simulink model "ControleNL_Degrau_2020a"  (R2020a)
settings: Solver=FixedStepAuto  StartTime=0  StopTime=10  FixedStep=1e-3  RelTol=1e-3
values from neighbouring files (symbols this model uses):
  alpha = alpha_vec(l)    [kermani_parameters.m]    (also in teste_controle_nao_linear.m = 0.1)
  Fc = Fc_vec(k)    [kermani_parameters.m]    (also in teste_controle_nao_linear.m = 0.5)
  Fs = Fs_vec(j)    [kermani_parameters.m]    (also in teste_controle_nao_linear.m = 1.5)
  Jeff = 0.5    [kermani_parameters.m]    (also in teste_controle_nao_linear.m)
  K = (90/12)*(2*pi/60)    (= 0.785398163397)    [kermani_parameters.m]    (also in teste_controle_nao_linear.m)
  Kd = (2*xi*wn*Jeff - Beff)/K    (= 17.8253536263)    [kermani_parameters.m]    (also in teste_controle_nao_linear.m = -44.5633840657)
  Kp = (wn^2*Jeff)/K    (= 143.239448783)    [kermani_parameters.m]    (also in teste_controle_nao_linear.m)
  N = 3    [kermani_parameters.m]    (also in teste_controle_nao_linear.m)
  r = 1./[231.22*4 139.138 139.138 231.22 231.22]    [kermani_parameters.m]    (also in teste_controle_nao_linear.m)
  sigma0 = sigma0_vec(m)    [kermani_parameters.m]    (also in teste_controle_nao_linear.m = 10000)
  sigma1 = sigma1_vec(n)    [kermani_parameters.m]    (also in teste_controle_nao_linear.m = 500)
  sigma2 = sigma2_vec(o)    [kermani_parameters.m]    (also in teste_controle_nao_linear.m = 50)
libraries: simulink_extras x5
(part 1 of 2)
settings Model: Creator=Karoline  LastModifiedBy=lunet
settings DataIOCC: ReturnWorkspaceOutputs=off
settings DebuggingCC: ArithmeticOperatorsInVariantConditions=warning
settings SFSimCC: SimUseLocalCustomCode=off  CustomCodeUndefinedFunction=UseInterfaceOnly
settings RTWCC: RTWUseLocalCustomCode=off
settings CodeAppCC: StateflowObjectComments=on

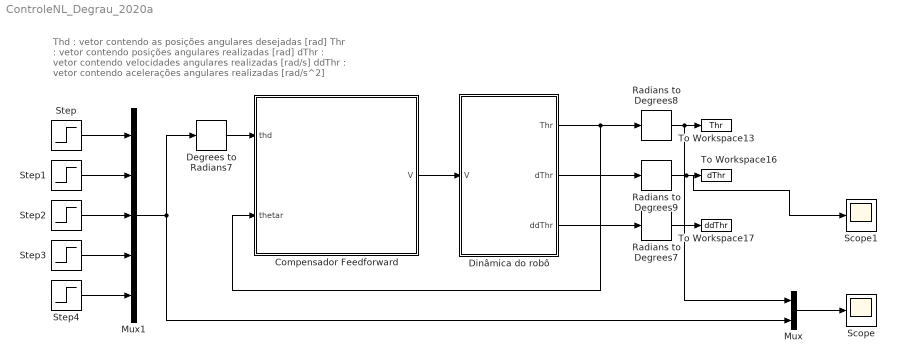
== system ControleNL_Degrau_2020a ==
  note: Thd : vetor contendo as posições angulares desejadas [rad]
      | Thr : vetor contendo posições angulares realizadas [rad]
      | dThr : vetor contendo velocidades angulares realizadas [rad/s]
      | ddThr : vetor contendo acelerações angulares realizadas [rad/s^2]
  Compensador Feedforward : Subsystem
  Degrees to Radians7 : simulink_extras/Transformations/Degrees to Radians
  Dinâmica do robô : Subsystem
  Mux : Mux  Inputs=2
  Mux1 : Mux  Inputs=5
  Radians to Degrees7 : simulink_extras/Transformations/Radians to Degrees
  Radians to Degrees8 : simulink_extras/Transformations/Radians to Degrees
  Radians to Degrees9 : simulink_extras/Transformations/Radians to Degrees
  Scope : Scope
  Scope1 : Scope
  Step : Step  After=10  SampleTime=0
  Step{1..4} (4 alike) : Step  After=0  SampleTime=0
  To Workspace13 : ToWorkspace  VariableName=Thr  SaveFormat=Structure With Time  SampleTime=-1
  To Workspace16 : ToWorkspace  VariableName=dThr  SaveFormat=Structure With Time  SampleTime=-1
  To Workspace17 : ToWorkspace  VariableName=ddThr  SaveFormat=Structure With Time  SampleTime=-1
  wires:
  Radians to Degrees9/1 -> Scope1/1, To Workspace16/1
  Radians to Degrees8/1 -> Mux/1, To Workspace13/1
  Radians to Degrees7/1 -> To Workspace17/1
  Dinâmica do robô/3(ddThr) -> Radians to Degrees7/1
  Dinâmica do robô/1(Thr) -> Compensador Feedforward/2(thetar), Radians to Degrees8/1
  Compensador Feedforward/1(V) -> Dinâmica do robô/1(V)
  Degrees to Radians7/1 -> Compensador Feedforward/1(thd)
  Dinâmica do robô/2("dThr ") -> Radians to Degrees9/1
  Mux/1 -> Scope/1
  Step/1 -> Mux1/1
  Step1/1 -> Mux1/2
  Step2/1 -> Mux1/3
  Step3/1 -> Mux1/4
  Step4/1 -> Mux1/5
  Mux1/1 -> Mux/2, Degrees to Radians7/1

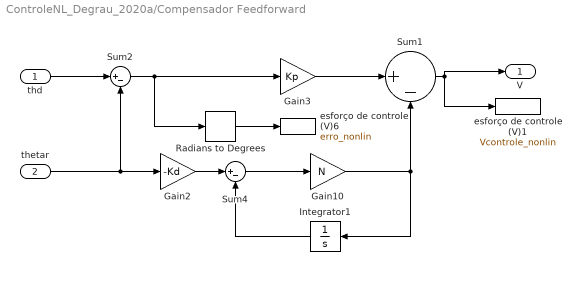
== system ControleNL_Degrau_2020a/Compensador Feedforward ==
  thd : Inport
  thetar : Inport  Port=2
  Gain10 : Gain  Gain=N
  Gain2 : Gain  Gain=-Kd
  Gain3 : Gain  Gain=Kp
  Integrator1 : Integrator
  Radians to Degrees : simulink_extras/Transformations/Radians to Degrees
  Sum1 : Sum  Inputs=|+-
  Sum2 : Sum  Inputs=|+-
  Sum4 : Sum  Inputs=|+-
  esforço de controle (V)1 : ToWorkspace  VariableName=Vcontrole_nonlin  SaveFormat=Structure With Time  SampleTime=-1
  esforço de controle (V)6 : ToWorkspace  VariableName=erro_nonlin  SaveFormat=Structure With Time  SampleTime=-1
  V : Outport  VectorParamsAs1DForOutWhenUnconnected=off
  wires:
  Gain2/1 -> Sum4/1
  thetar/1 -> Sum2/2, Gain2/1
  Sum4/1 -> Gain10/1
  Integrator1/1 -> Sum4/2
  Gain10/1 -> Sum1/2, Integrator1/1
  thd/1 -> Sum2/1
  Gain3/1 -> Sum1/1
  Sum1/1 -> V/1, esforço de controle (V)1/1
  Radians to Degrees/1 -> esforço de controle (V)6/1
  Sum2/1 -> Radians to Degrees/1, Gain3/1

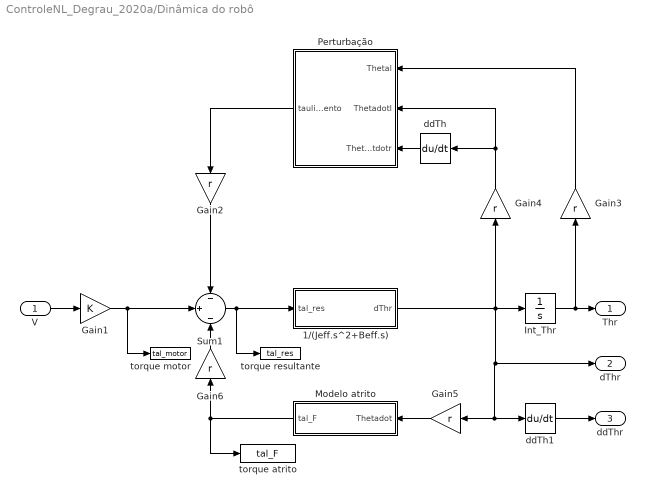
== system ControleNL_Degrau_2020a/Dinâmica do robô ==
  V : Inport
  1/(Jeff.s^2+Beff.s) : Subsystem
  Gain1 : Gain  Gain=K
  Gain{2..6} (5 alike) : Gain  Gain=r
  Int_Thr : Integrator  Tag=Int_Thr  InitialCondition=[0 0 0 0 0]
  Modelo atrito : Subsystem
  Perturbação : Subsystem
  Sum1 : Sum  Inputs=-|+|-
  ddTh : Derivative
  ddTh1 : Derivative
  torque atrito : ToWorkspace  VariableName=tal_F  SaveFormat=Structure With Time  SampleTime=-1
  torque motor : ToWorkspace  VariableName=tal_motor  SaveFormat=Structure With Time  SampleTime=-1
  torque resultante : ToWorkspace  VariableName=tal_res  SaveFormat=Structure With Time  SampleTime=-1
  Thr : Outport  VectorParamsAs1DForOutWhenUnconnected=off
  "dThr " : Outport  Port=2  VectorParamsAs1DForOutWhenUnconnected=off
  ddThr : Outport  Port=3  VectorParamsAs1DForOutWhenUnconnected=off
  wires:
  Perturbação/1(tauligamento) -> Gain2/1
  Gain1/1 -> torque motor/1, Sum1/2
  Int_Thr/1 -> Thr/1, Gain3/1
  V/1 -> Gain1/1
  Gain2/1 -> Sum1/1
  ddTh/1 -> Perturbação/3(Thetadotdotr)
  Gain3/1 -> Perturbação/1(Thetal)
  Gain4/1 -> ddTh/1, Perturbação/2(Thetadotl)
  Sum1/1 -> torque resultante/1, 1/(Jeff.s^2+Beff.s)/1(tal_res)
  ddTh1/1 -> ddThr/1
  1/(Jeff.s^2+Beff.s)/1(dThr) -> Gain5/1, ddTh1/1, "dThr "/1, Gain4/1, Int_Thr/1
  Modelo atrito/1(tal_F) -> torque atrito/1, Gain6/1
  Gain5/1 -> Modelo atrito/1(Thetadot)
  Gain6/1 -> Sum1/3

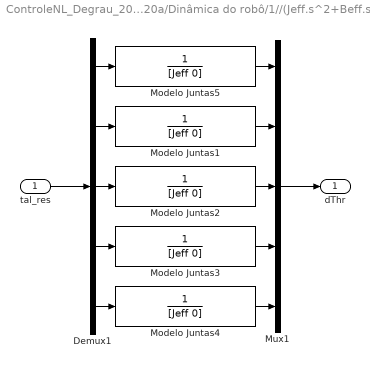
== system ControleNL_Degrau_2020a/Dinâmica do robô/1//(Jeff.s^2+Beff.s) ==
  tal_res : Inport
  Demux1 : Demux  Outputs=5
  Modelo Juntas{1..5} (5 alike) : TransferFcn  Denominator=[Jeff 0]
  Mux1 : Mux  Inputs=5
  dThr : Outport
  wires:
  Modelo Juntas5/1 -> Mux1/1
  Demux1/1 -> Modelo Juntas5/1
  Mux1/1 -> dThr/1
  tal_res/1 -> Demux1/1
  Demux1/2 -> Modelo Juntas1/1
  Modelo Juntas1/1 -> Mux1/2
  Demux1/5 -> Modelo Juntas4/1
  Demux1/4 -> Modelo Juntas3/1
  Demux1/3 -> Modelo Juntas2/1
  Modelo Juntas2/1 -> Mux1/3
  Modelo Juntas3/1 -> Mux1/4
  Modelo Juntas4/1 -> Mux1/5

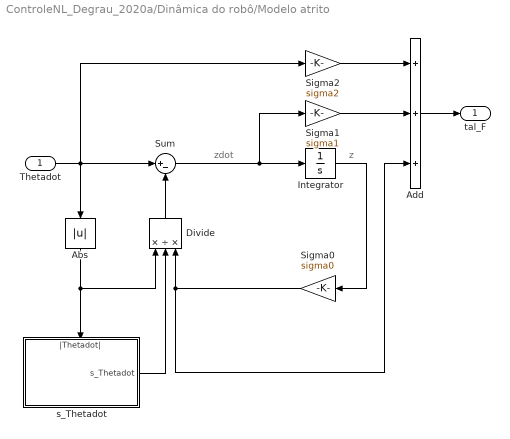
== system ControleNL_Degrau_2020a/Dinâmica do robô/Modelo atrito ==
  note: z
  note: zdot
  Thetadot : Inport
  Abs : Abs
  Add : Sum  Inputs=+++
  Divide : Product  Inputs=*/*
  Integrator : Integrator
  Sigma0 : Gain  Gain=sigma0
  Sigma1 : Gain  Gain=sigma1
  Sigma2 : Gain  Gain=sigma2
  Sum : Sum  Inputs=|+-
  s_Thetadot : Subsystem
      settings: PortSchema="{\"entries\":[{\"content\":{\"sides\":[{\"content\":{\"connectorIds\":[]},\"type\":\"ConnectorPlacement.EquallySpacedRectSide\",\"uuid\":\"4c4b190b-c928-4253-93d1-fd2ae137e0ab\"},{\"content\":{\"connectorIds\":[\"Out1\"],\"side\":\"RIGHT\"},\"type\":\"ConnectorPlacement.EquallySpacedRectSide\",\"uuid\":\"6a4109ad-b0a7-44dc-94f8-84112378c3da\"},{\"content\":{\"connectorIds\":[\"In1\"],\"side\":\"TOP\"},\"type\":\"ConnectorPlacement.EquallySpacedRectSide\",\"uuid\":\"364d9b06-17df-4fa5-ae25-87ed6816814d\"}]},\"type\":\"ConnectorPlacement.EquallySpacedConnector\",\"uuid\":\"c598e9c2-b687-45ab-b3d0-f2b281a49fb7\"}],\"packageUris\":[\"http://schema.mathworks.com/mf0/Connector/19700101\"],\"version\":\"1.0\"}"
  tal_F : Outport
  wires:
  Sigma0/1 -> Divide/3, Add/3
  Sigma1/1 -> Add/2
  Divide/1 -> Sum/2
  Abs/1 -> s_Thetadot/1(|Thetadot|), Divide/1
  s_Thetadot/1(s_Thetadot) -> Divide/2
  Sum/1 -> Sigma1/1, Integrator/1
  Thetadot/1 -> Sigma2/1, Sum/1, Abs/1
  Sigma2/1 -> Add/1
  Integrator/1 -> Sigma0/1
  Add/1 -> tal_F/1

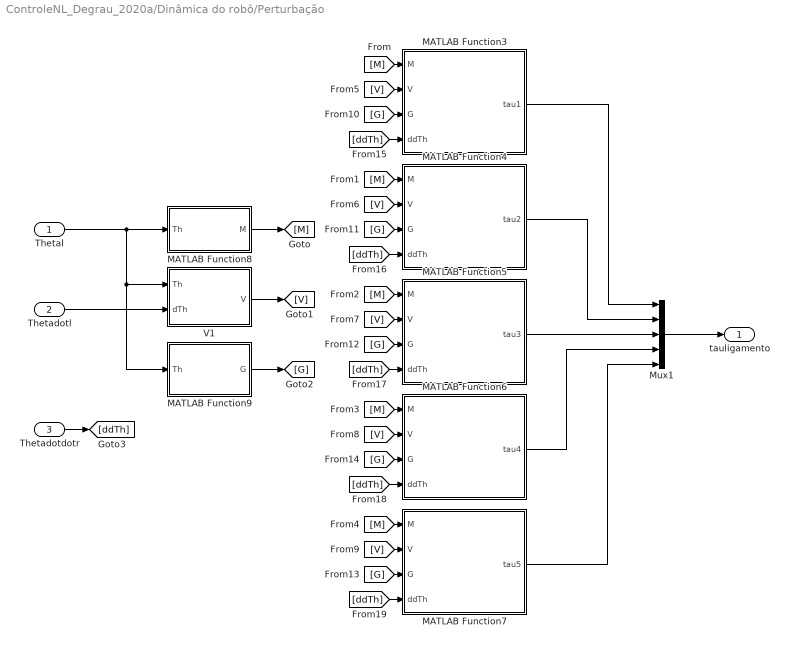
== system ControleNL_Degrau_2020a/Dinâmica do robô/Perturbação ==
  Thetal : Inport
  Thetadotl : Inport  Port=2
  Thetadotdotr : Inport  Port=3
  MATLAB Function3 : MATLAB Function  TreatAsAtomicUnit=on
  MATLAB Function4 : MATLAB Function  TreatAsAtomicUnit=on
  MATLAB Function5 : MATLAB Function  TreatAsAtomicUnit=on
  MATLAB Function6 : MATLAB Function  TreatAsAtomicUnit=on
  MATLAB Function7 : MATLAB Function  TreatAsAtomicUnit=on
  MATLAB Function8 : MATLAB Function  TreatAsAtomicUnit=on
  MATLAB Function9 : MATLAB Function  TreatAsAtomicUnit=on
  Mux1 : Mux  Inputs=5
  V1 : MATLAB Function  TreatAsAtomicUnit=on
  tauligamento : Outport  VectorParamsAs1DForOutWhenUnconnected=off
  wires:
  [G] -> MATLAB Function6/3(G)
  MATLAB Function8/1(M) -> [M]
  [M] -> MATLAB Function6/1(M)
  [M] -> MATLAB Function4/1(M)
  [M] -> MATLAB Function3/1(M)
  Thetal/1 -> MATLAB Function8/1(Th), MATLAB Function9/1(Th), V1/1(Th)
  [ddTh] -> MATLAB Function5/4(ddTh)
  [V] -> MATLAB Function3/2(V)
  [ddTh] -> MATLAB Function3/4(ddTh)
  [G] -> MATLAB Function7/3(G)
  [ddTh] -> MATLAB Function6/4(ddTh)
  [V] -> MATLAB Function6/2(V)
  Thetadotl/1 -> V1/2(dTh)
  [G] -> MATLAB Function5/3(G)
  [G] -> MATLAB Function3/3(G)
  [G] -> MATLAB Function4/3(G)
  MATLAB Function9/1(G) -> [G]
  [V] -> MATLAB Function7/2(V)
  [ddTh] -> MATLAB Function4/4(ddTh)
  [V] -> MATLAB Function5/2(V)
  [V] -> MATLAB Function4/2(V)
  V1/1(V) -> [V]
  [M] -> MATLAB Function7/1(M)
  [M] -> MATLAB Function5/1(M)
  [ddTh] -> MATLAB Function7/4(ddTh)
  Mux1/1 -> tauligamento/1
  MATLAB Function3/1(tau1) -> Mux1/1
  MATLAB Function4/1(tau2) -> Mux1/2
  MATLAB Function5/1(tau3) -> Mux1/3
  MATLAB Function6/1(tau4) -> Mux1/4
  MATLAB Function7/1(tau5) -> Mux1/5
  Thetadotdotr/1 -> [ddTh]

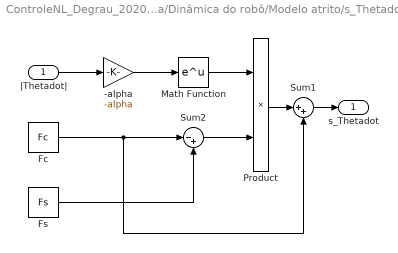
== system ControleNL_Degrau_2020a/Dinâmica do robô/Modelo atrito/s_Thetadot ==
  |Thetadot| : Inport
  -alpha : Gain  Gain=-alpha
  Fc : Constant  Value=Fc
  Fs : Constant  Value=Fs
  Math Function : Math  SaturateOnIntegerOverflow=on
  Product : Product
  Sum1 : Sum  Inputs=|++
  Sum2 : Sum  Inputs=|-+
  s_Thetadot : Outport
  wires:
  |Thetadot|/1 -> -alpha/1
  Fc/1 -> Sum2/1, Sum1/2
  -alpha/1 -> Math Function/1
  Sum1/1 -> s_Thetadot/1
  Fs/1 -> Sum2/2
  Math Function/1 -> Product/1
  Sum2/1 -> Product/2
  Product/1 -> Sum1/1

== matlab function ControleNL_Degrau_2020a/Dinâmica do robô/Perturbação/MATLAB Function3 ==
  data: M input; V input; tau1 output; G input; ddTh input
function tau1  = calcul_dk1(M, V, G, ddTh)

tau1 = M(1,2)*ddTh(2) + M(1,3)*ddTh(3) + M(1,4)*ddTh(4) + M(1,5)*ddTh(5) ...
       + V(1) + G(1);

== matlab function ControleNL_Degrau_2020a/Dinâmica do robô/Perturbação/MATLAB Function4 ==
  data: M input; V input; tau2 output; G input; ddTh input
function tau2  = calcul_dk2(M, V, G, ddTh)

tau2 = M(2,1)*ddTh(1) + M(2,3)*ddTh(3) + M(2,4)*ddTh(4) + M(2,5)*ddTh(5) ...
       + V(2) + G(2);

== matlab function ControleNL_Degrau_2020a/Dinâmica do robô/Perturbação/MATLAB Function5 ==
  data: M input; V input; tau3 output; G input; ddTh input
function tau3  = calcul_dk3(M, V, G, ddTh)

tau3 = M(3,1)*ddTh(1) + M(3,2)*ddTh(2) + M(3,4)*ddTh(4) + M(3,5)*ddTh(5) ...
       + V(3) + G(3);

== matlab function ControleNL_Degrau_2020a/Dinâmica do robô/Perturbação/MATLAB Function6 ==
  data: M input; V input; tau4 output; G input; ddTh input
function tau4 = calcul_dk4(M, V, G, ddTh)

tau4 = M(4,1)*ddTh(1) + M(4,2)*ddTh(2) + M(4,3)*ddTh(3) + M(4,5)*ddTh(5) ...
       + V(4) + G(4);

== matlab function ControleNL_Degrau_2020a/Dinâmica do robô/Perturbação/MATLAB Function7 ==
  data: M input; V input; tau5 output; G input; ddTh input
function tau5  = calcul_dk5(M, V, G, ddTh)

tau5 = M(5,1)*ddTh(1) + M(5,2)*ddTh(2) + M(5,3)*ddTh(3) + M(5,4)*ddTh(4) ...
       + V(5) + G(5);

== matlab function ControleNL_Degrau_2020a/Dinâmica do robô/Perturbação/MATLAB Function8 ==
  data: Th input; M output
function M = calcul_M(Th)

th1 = Th(1);
th2 = Th(2);
th3 = Th(3);
th4 = Th(4);
th5 = Th(5);

M = [ (87*cos(th2)^2*cos(th5))/2500 + (87*cos(th3)^2*cos(th5))/2500 - (33*cos(th2)^2*sin(th3))/50 + (53231*cos(th2)^2)/62500 + (8453*cos(th3)^2)/31250 - (9*cos(th5)^2)/3200 - (8453*cos(th2)^2*cos(th3)^2)/15625 - (217*cos(th2)^2*cos(th4)^2)/80000 + (9*cos(th2)^2*cos(th5)^2)/3200 - (217*cos(th3)^2*cos(th4)^2)/80000 + (9*cos(th3)^2*cos(th5)^2)/3200 - (87*cos(th2)^2*cos(th3)^2*cos(th5))/1250 - (33*cos(th2)*cos(th3)*sin(th2))/50 + (217*cos(th2)^2*cos(th3)^2*cos(th4)^2)/40000 - (9*cos(th2)^2*cos(th3)^2*cos(th5)^2)/1600 + (9*cos(th2)^2*cos(th4)^2*cos(th5)^2)/3200 + (9*cos(th3)^2*cos(th4)^2*cos(th5)^2)/3200 - (3*cos(th2)^2*cos(th5)*sin(th3))/80 - (9*cos(th2)^2*cos(th3)^2*cos(th4)^2*cos(th5)^2)/1600 - (3*cos(th2)*cos(th3)*cos(th5)*sin(th2))/80 + (8453*cos(th2)*cos(th3)*sin(th2)*sin(th3))/15625 - (87*cos(th2)*cos(th4)*sin(th2)*sin(th5))/2500 - (87*cos(th3)*cos(th4)*sin(th3)*sin(th5))/2500 - (3*cos(th2)^2*cos(th3)*cos(th4)*sin(th5))/80 + (3*cos(th2)*cos(th4)*sin(th2)*sin(th3)*sin(th5))/80 - (217*cos(th2)*cos(th3)*cos(th4)^2*sin(th2)*sin(th3))/40000 + (9*cos(th2)*cos(th3)*cos(th5)^2*sin(th2)*sin(th3))/1600 + (87*cos(th2)*cos(th3)^2*cos(th4)*sin(th2)*sin(th5))/1250 + (87*cos(th2)^2*cos(th3)*cos(th4)*sin(th3)*sin(th5))/1250 + (87*cos(th2)*cos(th3)*cos(th5)*sin(th2)*sin(th3))/1250 - (9*cos(th2)*cos(th4)*cos(th5)*sin(th2)*sin(th5))/1600 - (9*cos(th3)*cos(th4)*cos(th5)*sin(th3)*sin(th5))/1600 + (9*cos(th2)*cos(th3)*cos(th4)^2*cos(th5)^2*sin(th2)*sin(th3))/1600 + (9*cos(th2)*cos(th3)^2*cos(th4)*cos(th5)*sin(th2)*sin(th5))/800 + (9*cos(th2)^2*cos(th3)*cos(th4)*cos(th5)*sin(th3)*sin(th5))/800 + 3793/80000, -(sin(th4)*(1500*sin(th2)*sin(th5) - 217*cos(th2)*cos(th4)*sin(th3) - 217*cos(th3)*cos(th4)*sin(th2) + 1392*cos(th2)*cos(th3)*sin(th5) - 1392*sin(th2)*sin(th3)*sin(th5) + 225*cos(th2)*cos(th3)*cos(th5)*sin(th5) - 225*cos(th5)*sin(th2)*sin(th3)*sin(th5) + 225*cos(th2)*cos(th4)*cos(th5)^2*sin(th3) + 225*cos(th3)*cos(th4)*cos(th5)^2*sin(th2)))/80000, (sin(th4)*(217*cos(th2)*cos(th4)*sin(th3) + 217*cos(th3)*cos(th4)*sin(th2) - 1392*cos(th2)*cos(th3)*sin(th5) + 1392*sin(th2)*sin(th3)*sin(th5) - 225*cos(th2)*cos(th3)*cos(th5)*sin(th5) + 225*cos(th5)*sin(th2)*sin(th3)*sin(th5) - 225*cos(th2)*cos(th4)*cos(th5)^2*sin(th3) - 225*cos(th3)*cos(th4)*cos(th5)^2*sin(th2)))/80000, (489*cos(th2)*cos(th3))/80000 - (489*sin(th2)*sin(th3))/80000 - (3*cos(th2)*cos(th4)*sin(th5))/160 - (9*cos(th2)*cos(th3)*cos(th5)^2)/3200 + (9*cos(th5)^2*sin(th2)*sin(th3))/3200 + (87*cos(th2)*cos(th4)*sin(th3)*sin(th5))/5000 + (87*cos(th3)*cos(th4)*sin(th2)*sin(th5))/5000 + (9*cos(th2)*cos(th4)*cos(th5)*sin(th3)*sin(th5))/3200 + (9*cos(th3)*cos(th4)*cos(th5)*sin(th2)*sin(th5))/3200, (sin(th4)*(353*cos(th2)*sin(th3) + 353*cos(th3)*sin(th2) - 1500*cos(th2)*cos(th5) + 1392*cos(th2)*cos(th5)*sin(th3) + 1392*cos(th3)*cos(th5)*sin(th2)))/80000;
                                                                                                                                                                                                                                                                                                                                                                                                                                                                                                                                                                                                                                                                                                                                                                                                                                                                                                                                                                                                                                                                                                                                                                                                                                                                                                                                                                                                                                                                                                                                                                                            -(sin(th4)*(1500*sin(th2)*sin(th5) - 217*cos(th2)*cos(th4)*sin(th3) - 217*cos(th3)*cos(th4)*sin(th2) + 1392*cos(th2)*cos(th3)*sin(th5) - 1392*sin(th2)*sin(th3)*sin(th5) + 225*cos(th2)*cos(th3)*cos(th5)*sin(th5) - 225*cos(th5)*sin(th2)*sin(th3)*sin(th5) + 225*cos(th2)*cos(th4)*cos(th5)^2*sin(th3) + 225*cos(th3)*cos(th4)*cos(th5)^2*sin(th2)))/80000,                                                                                                                                                                                                                       (87*cos(th5))/2500 - (33*sin(th3))/50 - (3*cos(th5)*sin(th3))/80 + (217*cos(th4)^2)/80000 + (9*cos(th5)^2)/3200 - (9*cos(th4)^2*cos(th5)^2)/3200 - (3*cos(th3)*cos(th4)*sin(th5))/80 + 54781/62500,                                                                                                                                                                                   (87*cos(th5))/2500 - (33*sin(th3))/100 - (3*cos(th5)*sin(th3))/160 + (217*cos(th4)^2)/80000 + (9*cos(th5)^2)/3200 - (9*cos(th4)^2*cos(th5)^2)/3200 - (3*cos(th3)*cos(th4)*sin(th5))/160 + 72749/250000,                                                                                                                                                                                                                                                                                                                                                                                                                     -(3*sin(th4)*sin(th5)*(75*cos(th5) - 500*sin(th3) + 464))/80000,                                                          (353*cos(th4))/80000 - (3*cos(th3)*sin(th5))/160 + (87*cos(th4)*cos(th5))/5000 - (3*cos(th4)*cos(th5)*sin(th3))/160;
                                                                                                                                                                                                                                                                                                                                                                                                                                                                                                                                                                                                                                                                                                                                                                                                                                                                                                                                                                                                                                                                                                                                                                                                                                                                                                                                                                                                                                                                                                                                                                                                                            (sin(th4)*(217*cos(th2)*cos(th4)*sin(th3) + 217*cos(th3)*cos(th4)*sin(th2) - 1392*cos(th2)*cos(th3)*sin(th5) + 1392*sin(th2)*sin(th3)*sin(th5) - 225*cos(th2)*cos(th3)*cos(th5)*sin(th5) + 225*cos(th5)*sin(th2)*sin(th3)*sin(th5) - 225*cos(th2)*cos(th4)*cos(th5)^2*sin(th3) - 225*cos(th3)*cos(th4)*cos(th5)^2*sin(th2)))/80000,                                                                                                                                                                                                                   (87*cos(th5))/2500 - (33*sin(th3))/100 - (3*cos(th5)*sin(th3))/160 + (217*cos(th4)^2)/80000 + (9*cos(th5)^2)/3200 - (9*cos(th4)^2*cos(th5)^2)/3200 - (3*cos(th3)*cos(th4)*sin(th5))/160 + 72749/250000,                                                                                                                                                                                                                                                                                          (87*cos(th5))/2500 + (217*cos(th4)^2)/80000 + (9*cos(th5)^2)/3200 - (9*cos(th4)^2*cos(th5)^2)/3200 + 72749/250000,                                                                                                                                                                                                                                                                                                                                                                                                                                       -(3*sin(th4)*sin(th5)*(75*cos(th5) + 464))/80000,                                                                                                                                                         (cos(th4)*(1392*cos(th5) + 353))/80000;
                                                                                                                                                                                                                                                                                                                                                                                                                                                                                                                                                                                                                                                                                                                                                                                                                                                                                                                                                                                                                                                                                                                                                                                                                                                                                                                                                                                                                                                                                                                                                      (489*cos(th2)*cos(th3))/80000 - (489*sin(th2)*sin(th3))/80000 - (3*cos(th2)*cos(th4)*sin(th5))/160 - (9*cos(th2)*cos(th3)*cos(th5)^2)/3200 + (9*cos(th5)^2*sin(th2)*sin(th3))/3200 + (87*cos(th2)*cos(th4)*sin(th3)*sin(th5))/5000 + (87*cos(th3)*cos(th4)*sin(th2)*sin(th5))/5000 + (9*cos(th2)*cos(th4)*cos(th5)*sin(th3)*sin(th5))/3200 + (9*cos(th3)*cos(th4)*cos(th5)*sin(th2)*sin(th5))/3200,                                                                                                                                                                                                                                                                                                                                                                               -(3*sin(th4)*sin(th5)*(75*cos(th5) - 500*sin(th3) + 464))/80000,                                                                                                                                                                                                                                                                                                                                                                 -(3*sin(th4)*sin(th5)*(75*cos(th5) + 464))/80000,                                                                                                                                                                                                                                                                                                                                                                                                                                                              489/80000 - (9*cos(th5)^2)/3200,                                                                                                                                                                                                    0;
                                                                                                                                                                                                                                                                                                                                                                                                                                                                                                                                                                                                                                                                                                                                                                                                                                                                                                                                                                                                                                                                                                                                                                                                                                                                                                                                                                                                                                                                                                                                                                                                                                                                                                                                                                                                                                                 (sin(th4)*(353*cos(th2)*sin(th3) + 353*cos(th3)*sin(th2) - 1500*cos(th2)*cos(th5) + 1392*cos(th2)*cos(th5)*sin(th3) + 1392*cos(th3)*cos(th5)*sin(th2)))/80000,                                                                                                                                                                                                                                                                                                               (353*cos(th4))/80000 - (3*cos(th3)*sin(th5))/160 + (87*cos(th4)*cos(th5))/5000 - (3*cos(th4)*cos(th5)*sin(th3))/160,                                                                                                                                                                                                                                                                                                                                                                              (cos(th4)*(1392*cos(th5) + 353))/80000,                                                                                                                                                                                                                                                                                                                                                                                                                                                                                               0,                                                                                                                                                                                            353/80000];

== matlab function ControleNL_Degrau_2020a/Dinâmica do robô/Perturbação/MATLAB Function9 ==
  data: Th input; G output
function G = calcul_G(Th)

g = 9.80665;
th1 = Th(1);
th2 = Th(2);
th3 = Th(3);
th4 = Th(4);
th5 = Th(5);

G = [                                                                                                                                                                                                                                                                                               0;
 -g*((49*cos(th2)*sin(th3))/125 - cos(th2)/2 + (49*cos(th3)*sin(th2))/125 + (3*cos(th2)*cos(th5)*sin(th3))/40 + (3*cos(th3)*cos(th5)*sin(th2))/40 + (3*cos(th2)*cos(th3)*cos(th4)*sin(th5))/40 - (3*cos(th4)*sin(th2)*sin(th3)*sin(th5))/40);
                 -g*((49*cos(th2)*sin(th3))/125 + (49*cos(th3)*sin(th2))/125 + (3*cos(th2)*cos(th5)*sin(th3))/40 + (3*cos(th3)*cos(th5)*sin(th2))/40 + (3*cos(th2)*cos(th3)*cos(th4)*sin(th5))/40 - (3*cos(th4)*sin(th2)*sin(th3)*sin(th5))/40);
                                                                                                                                                                                                                                                (3*g*sin(th4)*sin(th5)*sin(th2 + th3))/40;
                                                                                       -g*((3*cos(th2)*cos(th3)*sin(th5))/40 - (3*sin(th2)*sin(th3)*sin(th5))/40 + (3*cos(th2)*cos(th4)*cos(th5)*sin(th3))/40 + (3*cos(th3)*cos(th4)*cos(th5)*sin(th2))/40)];
